simulink model "followerBlock"  (R2016a)
settings: Solver=VariableStepAuto  StartTime=0.0  StopTime=inf  RelTol=1e-3
undefined symbols (not defined in the file or in its folder): Angular, Linear
libraries: robotlib x6, simulink x1
settings Model: Creator=ece446  LastModifiedBy=ece446

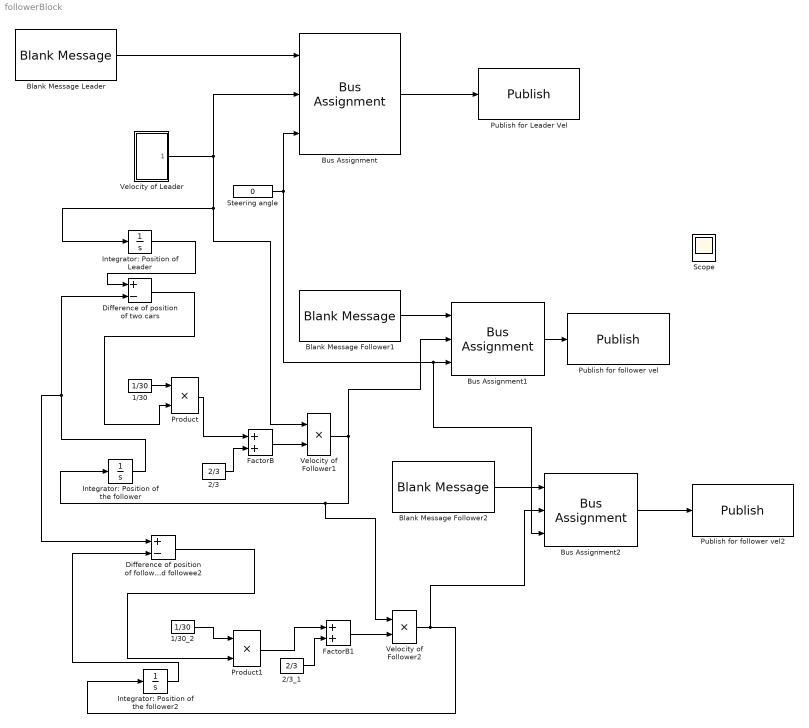
== system followerBlock ==
  1/30 : Constant  Value=1/30
  1/30_2 : Constant  Value=1/30
  2/3 : Constant  Value=2/3
  2/3_1 : Constant  Value=2/3
  Blank Message Follower1 : robotlib/Blank Message  SourceLibraryInfo=This block requires Robotics System Toolbox  messageType=geometry_msgs/Twist  SampleTime=inf
  Blank Message Follower2 : robotlib/Blank Message  SourceLibraryInfo=This block requires Robotics System Toolbox  messageType=geometry_msgs/Twist  SampleTime=inf
  Blank Message Leader : robotlib/Blank Message  SourceLibraryInfo=This block requires Robotics System Toolbox  messageType=geometry_msgs/Twist  SampleTime=inf
  Bus Assignment : BusAssignment  AssignedSignals=Linear.X,Angular.Z
  Bus Assignment1 : BusAssignment  AssignedSignals=Linear.X,Angular.Z
  Bus Assignment2 : BusAssignment  AssignedSignals=Linear.X,Angular.Z
  Difference of position of follower1 and followee2 : Sum  Inputs=+-
  Difference of position of two cars : Sum  Inputs=+-
  FactorB : Sum
  FactorB1 : Sum
  Integrator: Position of Leader : Integrator
  Integrator: Position of the follower : Integrator
  Integrator: Position of the follower2 : Integrator
  Product : Product
  Product1 : Product
  Publish for Leader Vel : robotlib/Publish  SourceLibraryInfo=This block requires Robotics System Toolbox  topicSource=Select from ROS network  topic=/azcar_sim/cmd_vel  messageType=geometry_msgs/Twist  messageQueueLength=1
  Publish for follower vel : robotlib/Publish  SourceLibraryInfo=This block requires Robotics System Toolbox  topicSource=Select from ROS network  topic=/follower_sim/cmd_vel  messageType=geometry_msgs/Twist  messageQueueLength=1
  Publish for follower vel2 : robotlib/Publish  SourceLibraryInfo=This block requires Robotics System Toolbox  topicSource=Specify your own  topic=/follower_sim2/cmd_vel  messageType=geometry_msgs/Twist  messageQueueLength=1
  "Scope " : Scope  NumInputPorts=2
  Steering angle : Constant  Value=0
  Velocity of Follower1 : Product
  Velocity of Follower2 : Product
  Velocity of Leader : Subsystem
  wires:
  Blank Message Leader/1 -> Bus Assignment/1
  Bus Assignment/1 -> Publish for Leader Vel/1
  1/30/1 -> Product/1
  Product/1 -> FactorB/1
  2/3/1 -> FactorB/2
  Blank Message Follower1/1 -> Bus Assignment1/1
  Bus Assignment1/1 -> Publish for follower vel/1
  Velocity of Follower1/1 -> Velocity of Follower2/1, Integrator: Position of the follower/1, Bus Assignment1/2
  FactorB/1 -> Velocity of Follower1/2
  Velocity of Leader/1(Velocity) -> Velocity of Follower1/1, Integrator: Position of Leader/1, Bus Assignment/2
  Difference of position of two cars/1 -> Product/2
  Integrator: Position of Leader/1 -> Difference of position of two cars/1
  Steering angle/1 -> Bus Assignment2/3, Bus Assignment1/3, Bus Assignment/3
  Blank Message Follower2/1 -> Bus Assignment2/1
  Bus Assignment2/1 -> Publish for follower vel2/1
  Integrator: Position of the follower/1 -> Difference of position of follower1 and followee2/1, Difference of position of two cars/2
  1/30_2/1 -> Product1/1
  Product1/1 -> FactorB1/1
  Difference of position of follower1 and followee2/1 -> Product1/2
  2/3_1/1 -> FactorB1/2
  FactorB1/1 -> Velocity of Follower2/2
  Integrator: Position of the follower2/1 -> Difference of position of follower1 and followee2/2
  Velocity of Follower2/1 -> Bus Assignment2/2, Integrator: Position of the follower2/1

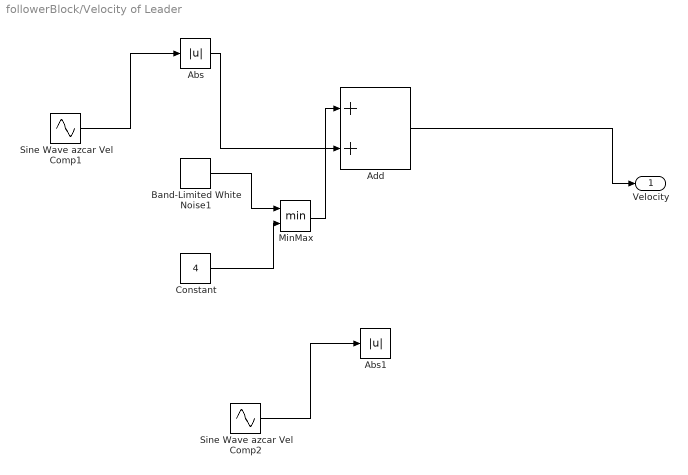
== system followerBlock/Velocity of Leader ==
  Abs : Abs
  Abs1 : Abs
  Add : Sum
  Band-Limited White Noise1 : simulink/Sources/Band-Limited White Noise  Cov=5  Ts=0.1  seed=[5]
  Constant : Constant  Value=4
  MinMax : MinMax  Inputs=2
  Sine Wave azcar Vel Comp1 : Sin  Amplitude=5  Frequency=3  SampleTime=0
  Sine Wave azcar Vel Comp2 : Sin  Amplitude=5  Frequency=3  SampleTime=0
  Velocity : Outport
  wires:
  Sine Wave azcar Vel Comp1/1 -> Abs/1
  Band-Limited White Noise1/1 -> MinMax/1
  Abs/1 -> Add/2
  Constant/1 -> MinMax/2
  MinMax/1 -> Add/1
  Sine Wave azcar Vel Comp2/1 -> Abs1/1
  Add/1 -> Velocity/1
